simulink subsystem "Poly_AeroProp"  (R2024b)
settings: Solver=VariableStepAuto  StartTime=0.0  StopTime=10.0  RelTol=1e-3
undefined symbols (not defined in the file or in its folder): SimIn
settings Model: Creator=macheson  LastModifiedBy=macheson

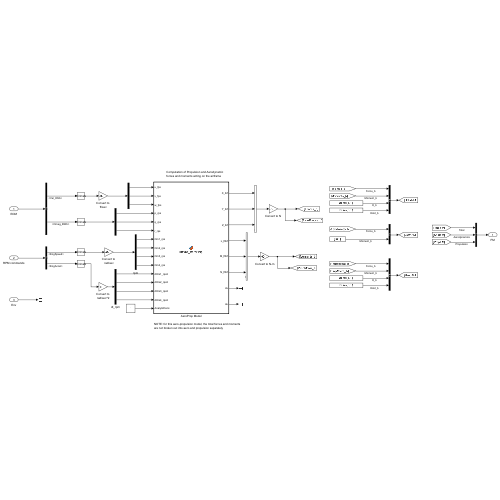
[thumbnail: Simulink's stored preview of the top-level diagram]
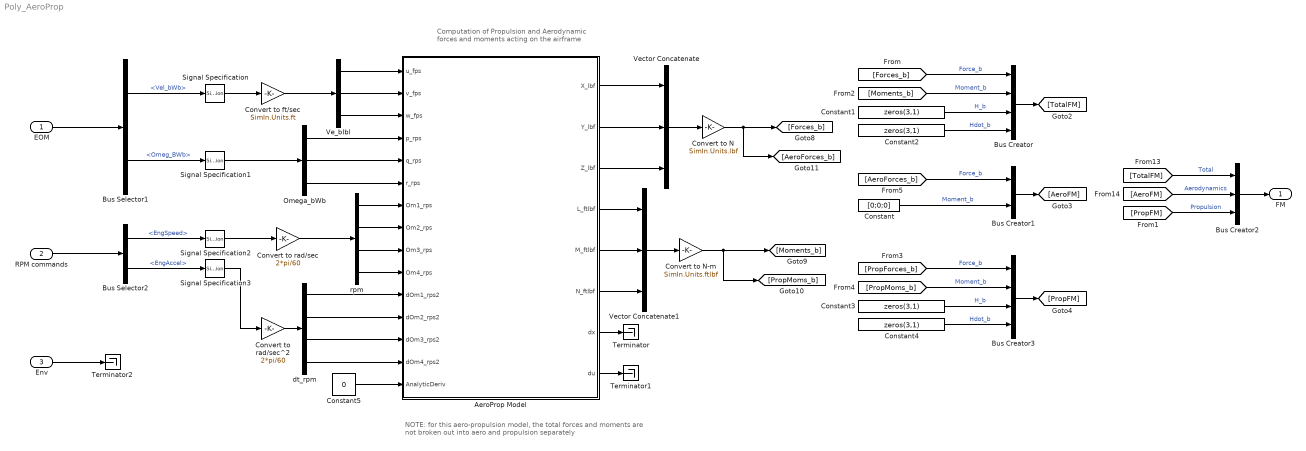
== system Poly_AeroProp ==
  note: Computation of Propulsion and Aerodynamic
      | forces and moments acting on the airframe
  note: NOTE: for this aero-propulsion model, the total forces and moments
      | are not broken out into aero and propulsion separately
  EOM : Inport
  RPM commands : Inport  Port=2
  Env : Inport  Port=3
  AeroProp Model : MATLAB Function  TreatAsAtomicUnit=on
  Bus Creator : BusCreator  Inputs=4
  Bus Creator1 : BusCreator  Inputs=2
  Bus Creator2 : BusCreator  Inputs=3  OutDataTypeStr=Bus: BUS_FORCE_MOMENT
  Bus Creator3 : BusCreator  Inputs=4
  Bus Selector1 : BusSelector  OutputSignals=AirRelativeData.Vel_bWb,AirRelativeData.Omeg_BWb
  Bus Selector2 : BusSelector  OutputSignals=EngSpeed,EngAccel
  Constant : Constant  Value=[0;0;0]  VectorParams1D=off
  Constant{1..4} (4 alike) : Constant  Value=zeros(3,1)  VectorParams1D=off
  Constant5 : Constant  Value=0
  Convert to ft/sec : Gain  Gain=SimIn.Units.ft
  Convert to rad/sec : Gain  Gain=2*pi/60
  Convert to rad/sec^2 : Gain  Gain=2*pi/60
  "Convert to N " : Gain  Gain=SimIn.Units.lbf
  Convert to N-m : Gain  Gain=SimIn.Units.ftlbf
  Omega_bWb : Demux  Outputs=3
  Signal Specification : SignalSpecification  Dimensions=3
  Signal Specification1 : SignalSpecification  Dimensions=3
  Signal Specification2 : SignalSpecification  Dimensions=4
  Signal Specification3 : SignalSpecification  Dimensions=4
  Terminator : Terminator
  Terminator1 : Terminator
  Terminator2 : Terminator
  Ve_bIbl : Demux  Outputs=3
  Vector Concatenate : Concatenate  NumInputs=3  Mode=Multidimensional array
  Vector Concatenate1 : Concatenate  NumInputs=3  Mode=Multidimensional array
  dt_rpm : Demux
  rpm : Demux
  FM : Outport  VectorParamsAs1DForOutWhenUnconnected=off
  wires:
  [TotalFM] -> Bus Creator2/1  "Total"
  [AeroForces_b] -> Bus Creator1/1  "Force_b"
  Constant4/1 -> Bus Creator3/4  "Hdot_b"
  [Moments_b] -> Bus Creator/2  "Moment_b"
  Constant1/1 -> Bus Creator/3  "H_b"
  Constant2/1 -> Bus Creator/4  "Hdot_b"
  Bus Creator/1 -> [TotalFM]
  Constant/1 -> Bus Creator1/2  "Moment_b"
  Constant3/1 -> Bus Creator3/3  "H_b"
  [Forces_b] -> Bus Creator/1  "Force_b"
  [AeroFM] -> Bus Creator2/2  "Aerodynamics"
  Bus Creator2/1 -> FM/1
  [PropMoms_b] -> Bus Creator3/2  "Moment_b"
  Bus Creator1/1 -> [AeroFM]
  [PropForces_b] -> Bus Creator3/1  "Force_b"
  [PropFM] -> Bus Creator2/3  "Propulsion"
  Bus Creator3/1 -> [PropFM]
  Constant5/1 -> AeroProp Model/15(AnalyticDeriv)
  AeroProp Model/1(X_lbf) -> Vector Concatenate/1
  AeroProp Model/2(Y_lbf) -> Vector Concatenate/2
  AeroProp Model/3(Z_lbf) -> Vector Concatenate/3
  AeroProp Model/4(L_ftlbf) -> Vector Concatenate1/1
  AeroProp Model/5(M_ftlbf) -> Vector Concatenate1/2
  AeroProp Model/6(N_ftlbf) -> Vector Concatenate1/3
  AeroProp Model/7(dx) -> Terminator/1
  AeroProp Model/8(du) -> Terminator1/1
  Vector Concatenate/1 -> "Convert to N "/1
  Vector Concatenate1/1 -> Convert to N-m/1
  Bus Selector1/2 -> Signal Specification1/1  "<Omeg_BWb>"
  EOM/1 -> Bus Selector1/1
  Bus Selector1/1 -> Signal Specification/1  "<Vel_bWb>"
  Convert to ft/sec/1 -> Ve_bIbl/1
  Omega_bWb/1 -> AeroProp Model/4(p_rps)
  Omega_bWb/2 -> AeroProp Model/5(q_rps)
  Omega_bWb/3 -> AeroProp Model/6(r_rps)
  Ve_bIbl/1 -> AeroProp Model/1(u_fps)
  Ve_bIbl/2 -> AeroProp Model/2(v_fps)
  Ve_bIbl/3 -> AeroProp Model/3(w_fps)
  Bus Selector2/1 -> Signal Specification2/1  "<EngSpeed>"
  RPM commands/1 -> Bus Selector2/1
  rpm/1 -> AeroProp Model/7(Om1_rps)
  rpm/2 -> AeroProp Model/8(Om2_rps)
  rpm/3 -> AeroProp Model/9(Om3_rps)
  rpm/4 -> AeroProp Model/10(Om4_rps)
  dt_rpm/4 -> AeroProp Model/14(dOm4_rps2)
  dt_rpm/3 -> AeroProp Model/13(dOm3_rps2)
  dt_rpm/2 -> AeroProp Model/12(dOm2_rps2)
  dt_rpm/1 -> AeroProp Model/11(dOm1_rps2)
  Bus Selector2/2 -> Signal Specification3/1  "<EngAccel>"
  Signal Specification/1 -> Convert to ft/sec/1
  Signal Specification1/1 -> Omega_bWb/1
  Signal Specification2/1 -> Convert to rad/sec/1
  Signal Specification3/1 -> Convert to rad/sec^2/1
  Convert to rad/sec/1 -> rpm/1
  Convert to rad/sec^2/1 -> dt_rpm/1
  "Convert to N "/1 -> [AeroForces_b], [Forces_b]
  Convert to N-m/1 -> [PropMoms_b], [Moments_b]
  Env/1 -> Terminator2/1

== matlab function Poly_AeroProp/AeroProp Model ==
  data: u_fps input; X_lbf output; v_fps input; w_fps input; p_rps input; q_rps input; r_rps input; Om1_rps input; Om2_rps input; Om3_rps input; Om4_rps input; dOm1_rps2 input; dOm2_rps2 input; dOm3_rps2 input; dOm4_rps2 input; AnalyticDeriv input; Y_lbf output; Z_lbf output; L_ftlbf output; M_ftlbf output; N_ftlbf output; dx output; du output
function [X_lbf,Y_lbf,Z_lbf,L_ftlbf,M_ftlbf,N_ftlbf, dx, du] = ...
        Impact_AeroProp(u_fps, v_fps, w_fps, p_rps, q_rps, r_rps, ... 
        Om1_rps, Om2_rps, Om3_rps, Om4_rps, ... 
        dOm1_rps2, dOm2_rps2, dOm3_rps2, dOm4_rps2, AnalyticDeriv)

    % Polynomial AeroProp modeling
    [X_lbf,Y_lbf,Z_lbf,L_ftlbf,M_ftlbf,N_ftlbf, dx, du] = ...
        IMPACT_AeroProp_RSE_V1_10Jun25_180239( ... 
        u_fps, v_fps, w_fps, p_rps, q_rps, r_rps, ... 
        Om1_rps, Om2_rps, Om3_rps, Om4_rps, ... 
        dOm1_rps2, dOm2_rps2, dOm3_rps2, dOm4_rps2, AnalyticDeriv);
